simulink model "Mathmatical_Equations_1"  (R2023b)
settings: Solver=VariableStepAuto  StartTime=0.0  StopTime=100.0  MaxStep=0.01  RelTol=1e-3
undefined symbols (not defined in the file): A, F, Ti

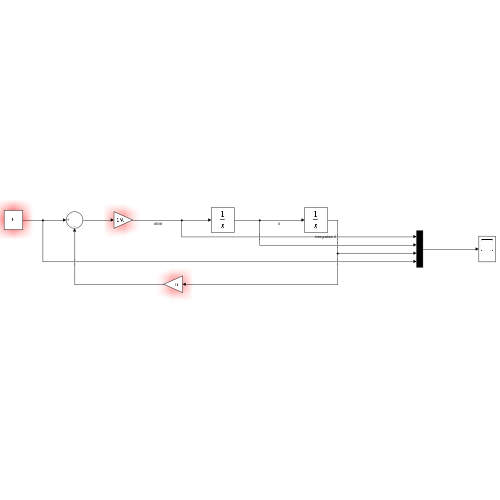
[thumbnail: Simulink's stored preview of the top-level diagram]
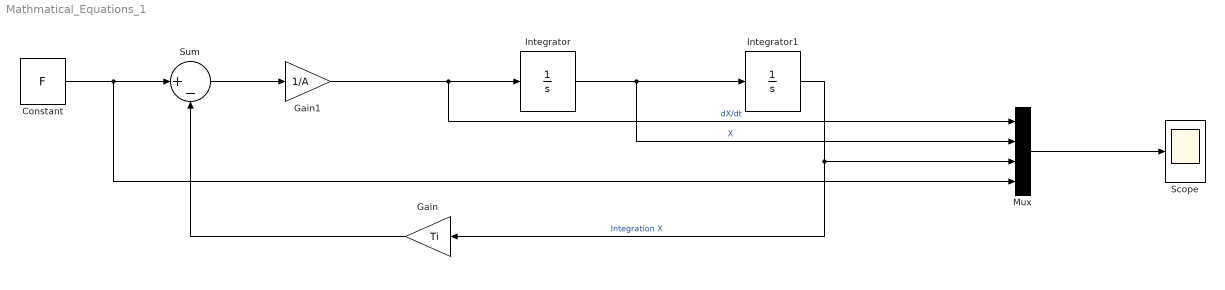
== system Mathmatical_Equations_1 ==
  Constant : Constant  Value=F
  Gain : Gain  Gain=Ti
  Gain1 : Gain  Gain=1/A
  Integrator : Integrator
  Integrator1 : Integrator
  Mux : Mux
  Scope : Scope
  Sum : Sum  Inputs=|+-
  wires:
  Integrator/1 -> Mux/2, Integrator1/1  "X"
  Constant/1 -> Mux/4, Sum/1
  Integrator1/1 -> Gain/1, Mux/3  "Integration X"
  Gain/1 -> Sum/2
  Sum/1 -> Gain1/1
  Gain1/1 -> Mux/1, Integrator/1  "dX/dt"
  Mux/1 -> Scope/1
